simulink model "stage1_encoder_model"  (R2026a)
settings: Solver=ode45  StopTime=0.5
undefined symbols (not defined in the file): B, CPR, J, Ke, Kt, L, R, TL
settings Model: Creator=knavn  LastModifiedBy=knavn

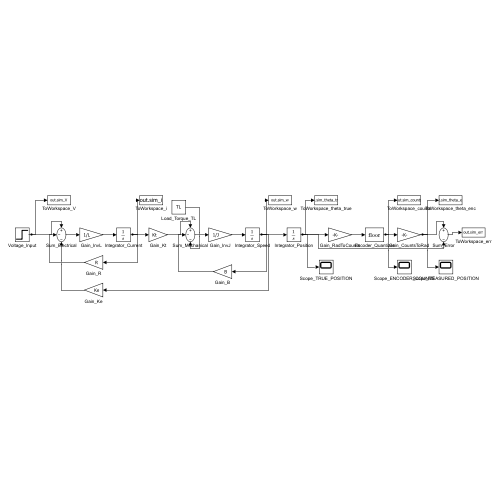
[thumbnail: Simulink's stored preview of the top-level diagram]
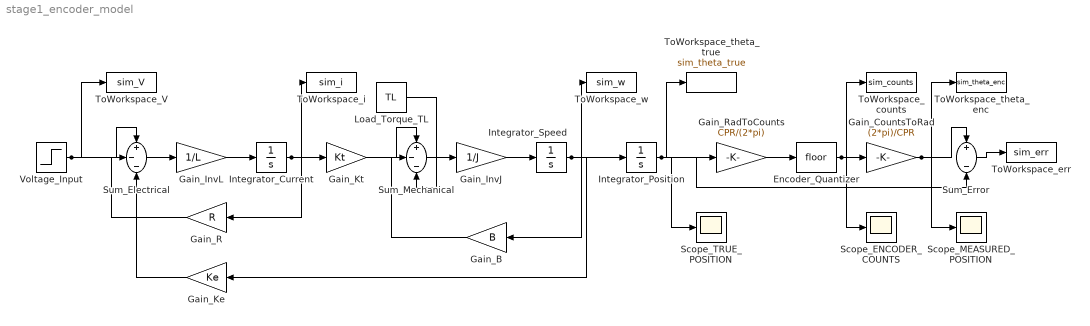
== system stage1_encoder_model ==
  Encoder_Quantizer : Rounding
  Gain_B : Gain  Gain=B
  Gain_CountsToRad : Gain  Gain=(2*pi)/CPR
  Gain_InvJ : Gain  Gain=1/J
  Gain_InvL : Gain  Gain=1/L
  Gain_Ke : Gain  Gain=Ke
  Gain_Kt : Gain  Gain=Kt
  Gain_R : Gain  Gain=R
  Gain_RadToCounts : Gain  Gain=CPR/(2*pi)
  Integrator_Current : Integrator
  Integrator_Position : Integrator
  Integrator_Speed : Integrator
  Load_Torque_TL : Constant  Value=TL
  Scope_ENCODER_COUNTS : Scope
  Scope_MEASURED_POSITION : Scope
  Scope_TRUE_POSITION : Scope
  Sum_Electrical : Sum  Inputs=+--
  Sum_Error : Sum  Inputs=+-
  Sum_Mechanical : Sum  Inputs=+--
  ToWorkspace_V : ToWorkspace  VariableName=sim_V  SaveFormat=Timeseries  SampleTime=-1
  ToWorkspace_counts : ToWorkspace  VariableName=sim_counts  SaveFormat=Timeseries  SampleTime=-1
  ToWorkspace_err : ToWorkspace  VariableName=sim_err  SaveFormat=Timeseries  SampleTime=-1
  ToWorkspace_i : ToWorkspace  VariableName=sim_i  SaveFormat=Timeseries  SampleTime=-1
  ToWorkspace_theta_enc : ToWorkspace  VariableName=sim_theta_enc  SaveFormat=Timeseries  SampleTime=-1
  ToWorkspace_theta_true : ToWorkspace  VariableName=sim_theta_true  SaveFormat=Timeseries  SampleTime=-1
  ToWorkspace_w : ToWorkspace  VariableName=sim_w  SaveFormat=Timeseries  SampleTime=-1
  Voltage_Input : Step  Time=0.05  FinalValue=12  SampleTime=0
  wires:
  Voltage_Input/1 -> Sum_Electrical/1, ToWorkspace_V/1
  Sum_Electrical/1 -> Gain_InvL/1
  Gain_InvL/1 -> Integrator_Current/1
  Integrator_Current/1 -> Gain_R/1, Gain_Kt/1, ToWorkspace_i/1
  Gain_R/1 -> Sum_Electrical/2
  Gain_Kt/1 -> Sum_Mechanical/1
  Load_Torque_TL/1 -> Sum_Mechanical/3
  Sum_Mechanical/1 -> Gain_InvJ/1
  Gain_InvJ/1 -> Integrator_Speed/1
  Integrator_Speed/1 -> Gain_B/1, Gain_Ke/1, Integrator_Position/1, ToWorkspace_w/1
  Gain_B/1 -> Sum_Mechanical/2
  Gain_Ke/1 -> Sum_Electrical/3
  Integrator_Position/1 -> ToWorkspace_theta_true/1, Scope_TRUE_POSITION/1, Gain_RadToCounts/1, Sum_Error/2
  Gain_RadToCounts/1 -> Encoder_Quantizer/1
  Encoder_Quantizer/1 -> ToWorkspace_counts/1, Scope_ENCODER_COUNTS/1, Gain_CountsToRad/1
  Gain_CountsToRad/1 -> ToWorkspace_theta_enc/1, Scope_MEASURED_POSITION/1, Sum_Error/1
  Sum_Error/1 -> ToWorkspace_err/1
